simulink model "VIPL557TrgtPos"  (R2018b)
settings: Solver=FixedStepDiscrete  StartTime=0.0  StopTime=10.0  RelTol=1e-3
settings Model: ModifiedHistory=2024.6.28 V3.0.0 座椅模式流程图V1.9  Creator=sn2xws  LastModifiedBy=sn2xws
settings DataIOCC: SaveFormat=StructureWithTime
settings OptimizationCC: DefaultParameterBehavior=Inlined  EnhancedBackFolding=on  PassReuseOutputArgsAs=Individual arguments  ZeroExternalMemoryAtStartup=off  ZeroInternalMemoryAtStartup=off  OptimizeBlockOrder=speed  DifferentSizesBufferReuse=on  OptimizationCustomize=off
settings DebuggingCC: ParameterTunabilityLossMsg=error
settings SFSimCC: MATLABDynamicMemAlloc=off
settings RTWCC: SystemTargetFile=autosar.tlc  GenCodeOnly=on  TemplateMakefile=ert_default_tmf  Description=AUTOSAR  GenerateReport=on  IncludeHyperlinkInReport=on  LaunchReport=on  GenerateTraceInfo=on  GenerateTraceReport=on  GenerateTraceReportSl=on  GenerateTraceReportSf=on  GenerateTraceReportEml=on
settings CodeAppCC: ForceParamTrailComments=on  IgnoreCustomStorageClasses=off  OperatorAnnotations=on  SimulinkDataObjDesc=on  SFDataObjDesc=on  InsertBlockDesc=on
settings STFCustomTargetCC: TargetLangStandard=C99 (ISO)  MultiwordLength=256  ParMdlRefBuildCompliant=on  CompOptLevelCompliant=on  IncludeMdlTerminateFcn=off  CombineOutputUpdateFcns=on  SuppressErrorStatus=on  ERTCustomFileBanners=on  SupportNonFinite=off  SupportComplex=off  SupportContinuousTime=off  SupportNonInlinedSFcns=off  RemoveResetFunc=on  MATLABClassNameForMDSCustomization=Simulink.SoftwareTarget.ERTCustomization  AutosarCompliant=on  UseToolchainInfoCompliant=on  LookupTableObjectStructAxisOrder=2,1,3,4,...  LUTObjectStructOrderEvenSpacing=Size,Table,Breakpoints  SystemTargetFile=autosar.tlc
settings ERTTargetCC: TargetLangStandard=C99 (ISO)  ConcurrentExecutionCompliant=off  IncludeMdlTerminateFcn=off  SuppressErrorStatus=on  SupportNonFinite=off  SupportComplex=off  ModelStepFunctionPrototypeControlCompliant=off  CPPClassGenCompliant=off  AutosarCompliant=on  LookupTableObjectStructAxisOrder=2,1,3,4,...  LUTObjectStructOrderEvenSpacing=Size,Table,Breakpoints  InlinedParameterPlacement=NonHierarchical  ERTCustomFileTemplate=example_file_process.tlc  ERTFilePackagingFormat=Compact

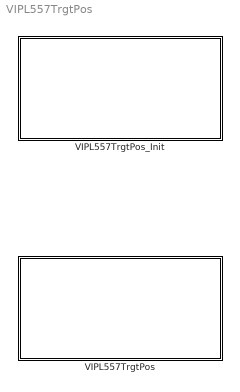
== system VIPL557TrgtPos ==
  VIPL557TrgtPos : Subsystem
  VIPL557TrgtPos_Init : Subsystem

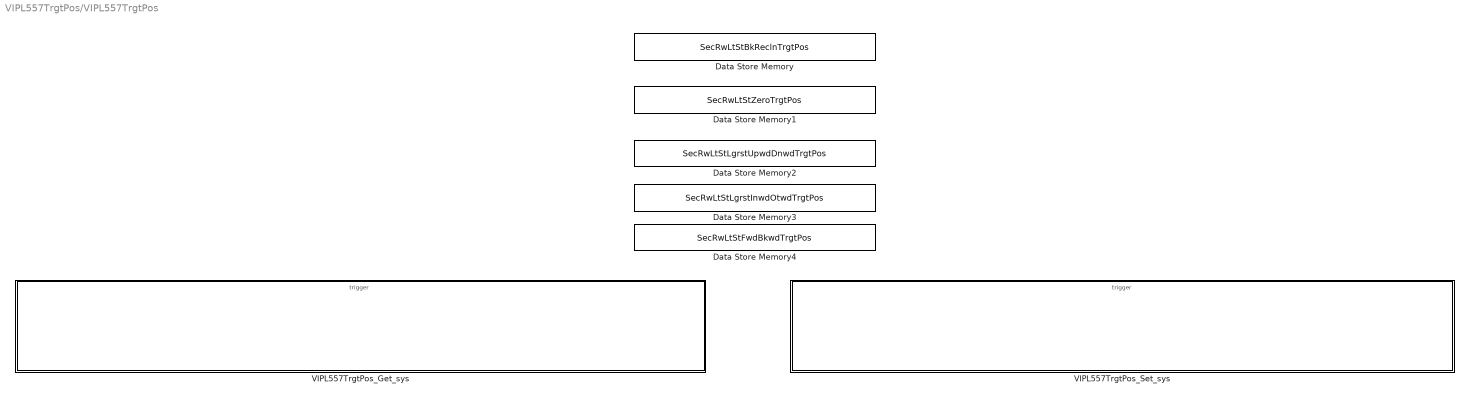
== system VIPL557TrgtPos/VIPL557TrgtPos ==
  Data Store Memory : DataStoreMemory  DataStoreName=SecRwLtStBkReclnTrgtPos  ReadBeforeWriteMsg=warning  WriteAfterWriteMsg=warning  WriteAfterReadMsg=warning  ShowAdditionalParam=off
  Data Store Memory1 : DataStoreMemory  DataStoreName=SecRwLtStZeroTrgtPos  ReadBeforeWriteMsg=warning  WriteAfterWriteMsg=warning  WriteAfterReadMsg=warning  ShowAdditionalParam=off
  Data Store Memory2 : DataStoreMemory  DataStoreName=SecRwLtStLgrstUpwdDnwdTrgtPos  ReadBeforeWriteMsg=warning  WriteAfterWriteMsg=warning  WriteAfterReadMsg=warning  ShowAdditionalParam=off
  Data Store Memory3 : DataStoreMemory  DataStoreName=SecRwLtStLgrstInwdOtwdTrgtPos  ReadBeforeWriteMsg=warning  WriteAfterWriteMsg=warning  WriteAfterReadMsg=warning  ShowAdditionalParam=off
  Data Store Memory4 : DataStoreMemory  DataStoreName=SecRwLtStFwdBkwdTrgtPos  ReadBeforeWriteMsg=warning  WriteAfterWriteMsg=warning  WriteAfterReadMsg=warning  ShowAdditionalParam=off
  VIPL557TrgtPos_Get_sys : Subsystem
  VIPL557TrgtPos_Set_sys : Subsystem

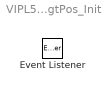
== system VIPL557TrgtPos/VIPL557TrgtPos_Init ==
  Event Listener : EventListener  EventName=reset

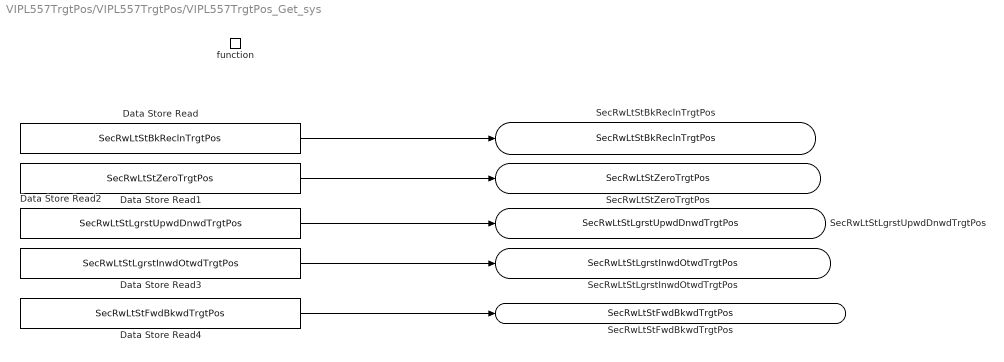
== system VIPL557TrgtPos/VIPL557TrgtPos/VIPL557TrgtPos_Get_sys ==
  function : TriggerPort  TriggerType=function-call  IsSimulinkFunction=on  FunctionName=VIPL557TrgtPos_Get  VariantControl=(inherit)
  Data Store Read : DataStoreRead  DataStoreName=SecRwLtStBkReclnTrgtPos
  Data Store Read1 : DataStoreRead  DataStoreName=SecRwLtStZeroTrgtPos
  Data Store Read2 : DataStoreRead  DataStoreName=SecRwLtStLgrstUpwdDnwdTrgtPos
  Data Store Read3 : DataStoreRead  DataStoreName=SecRwLtStLgrstInwdOtwdTrgtPos
  Data Store Read4 : DataStoreRead  DataStoreName=SecRwLtStFwdBkwdTrgtPos
  SecRwLtStBkReclnTrgtPos : ArgOut  OutDataTypeStr=uint16  ArgumentName=SecRwLtStBkReclnTrgtPos
  SecRwLtStZeroTrgtPos : ArgOut  Port=2  OutDataTypeStr=uint16  ArgumentName=SecRwLtStZeroTrgtPos
  SecRwLtStLgrstUpwdDnwdTrgtPos : ArgOut  Port=3  OutDataTypeStr=uint16  ArgumentName=SecRwLtStLgrstUpwdDnwdTrgtPos
  SecRwLtStLgrstInwdOtwdTrgtPos : ArgOut  Port=4  OutDataTypeStr=uint16  ArgumentName=SecRwLtStLgrstInwdOtwdTrgtPos
  SecRwLtStFwdBkwdTrgtPos : ArgOut  Port=5  OutDataTypeStr=uint16  ArgumentName=SecRwLtStFwdBkwdTrgtPos
  wires:
  Data Store Read/1 -> SecRwLtStBkReclnTrgtPos/1
  Data Store Read1/1 -> SecRwLtStZeroTrgtPos/1
  Data Store Read2/1 -> SecRwLtStLgrstUpwdDnwdTrgtPos/1
  Data Store Read3/1 -> SecRwLtStLgrstInwdOtwdTrgtPos/1
  Data Store Read4/1 -> SecRwLtStFwdBkwdTrgtPos/1

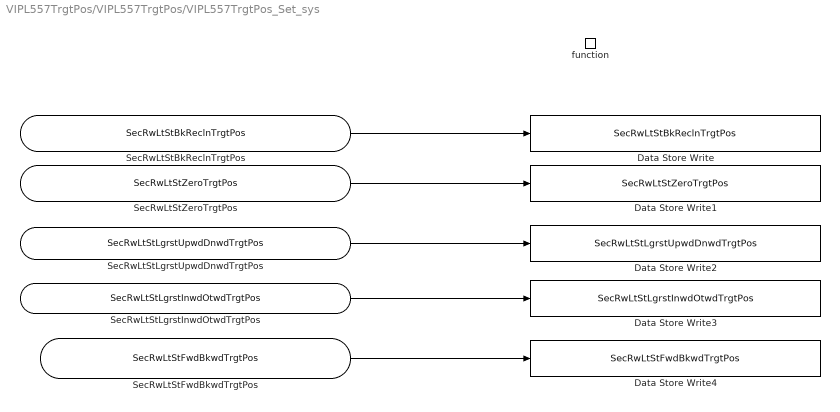
== system VIPL557TrgtPos/VIPL557TrgtPos/VIPL557TrgtPos_Set_sys ==
  function : TriggerPort  TriggerType=function-call  IsSimulinkFunction=on  FunctionName=VIPL557TrgtPos_Set  VariantControl=(inherit)
  Data Store Write : DataStoreWrite  DataStoreName=SecRwLtStBkReclnTrgtPos
  Data Store Write1 : DataStoreWrite  DataStoreName=SecRwLtStZeroTrgtPos
  Data Store Write2 : DataStoreWrite  DataStoreName=SecRwLtStLgrstUpwdDnwdTrgtPos
  Data Store Write3 : DataStoreWrite  DataStoreName=SecRwLtStLgrstInwdOtwdTrgtPos
  Data Store Write4 : DataStoreWrite  DataStoreName=SecRwLtStFwdBkwdTrgtPos
  SecRwLtStBkReclnTrgtPos : ArgIn  OutDataTypeStr=uint16  ArgumentName=SecRwLtStBkReclnTrgtPos
  SecRwLtStZeroTrgtPos : ArgIn  Port=2  OutDataTypeStr=uint16  ArgumentName=SecRwLtStZeroTrgtPos
  SecRwLtStLgrstUpwdDnwdTrgtPos : ArgIn  Port=3  OutDataTypeStr=uint16  ArgumentName=SecRwLtStLgrstUpwdDnwdTrgtPos
  SecRwLtStLgrstInwdOtwdTrgtPos : ArgIn  Port=4  OutDataTypeStr=uint16  ArgumentName=SecRwLtStLgrstInwdOtwdTrgtPos
  SecRwLtStFwdBkwdTrgtPos : ArgIn  Port=5  OutDataTypeStr=uint16  ArgumentName=SecRwLtStFwdBkwdTrgtPos
  wires:
  SecRwLtStBkReclnTrgtPos/1 -> Data Store Write/1
  SecRwLtStZeroTrgtPos/1 -> Data Store Write1/1
  SecRwLtStLgrstInwdOtwdTrgtPos/1 -> Data Store Write3/1
  SecRwLtStLgrstUpwdDnwdTrgtPos/1 -> Data Store Write2/1
  SecRwLtStFwdBkwdTrgtPos/1 -> Data Store Write4/1
